simulink model "ABS_v1"  (R2022a)
settings: Solver=VariableStepAuto  StartTime=0.0  StopTime=50.0  RelTol=1e-3
InitFcn:
  | m=75;
  | g=9.81;
  | I=5;
  | R=2;
  | v0=100;
settings Model: Creator=DELL  LastModifiedBy=DELL

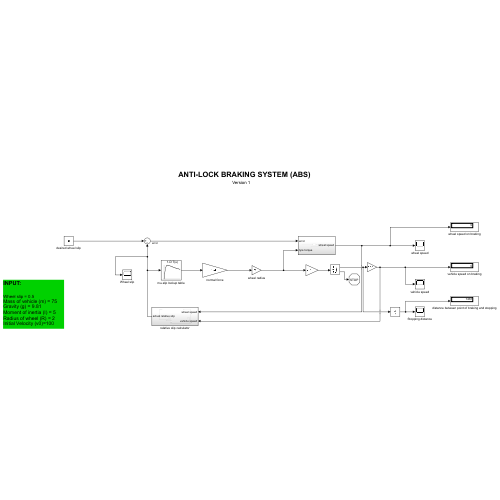
[thumbnail: Simulink's stored preview of the top-level diagram]
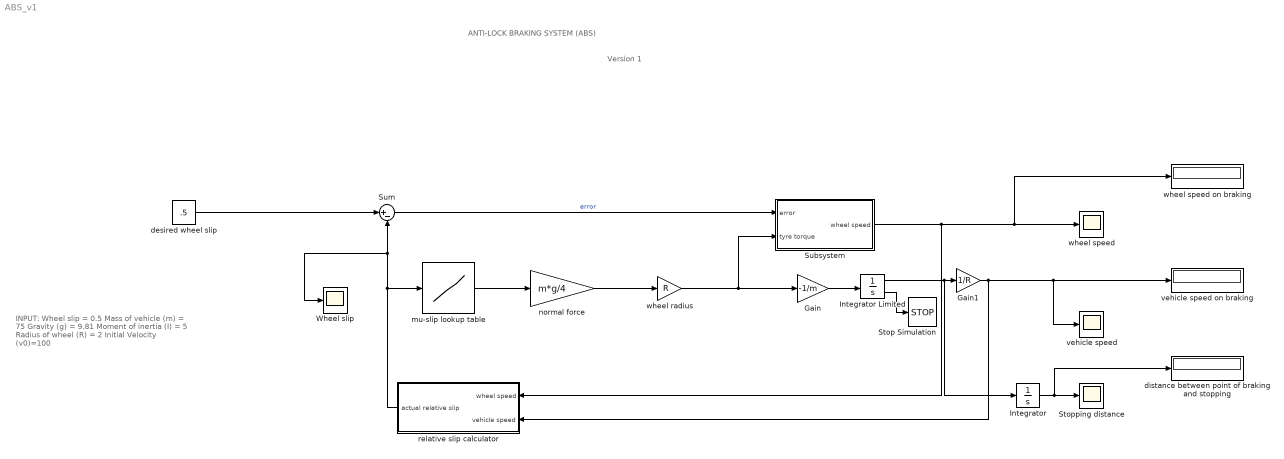
== system ABS_v1 ==
  note: INPUT:
      |
      | Wheel slip = 0.5
      | Mass of vehicle (m) = 75
      | Gravity (g) = 9.81
      | Moment of inertia (I) = 5
      | Radius of wheel (R) = 2
      | Initial Velocity (v0)=100
  note: Version 1
  note: ANTI-LOCK BRAKING SYSTEM (ABS)
  Gain : Gain  Gain=-1/m
  Gain1 : Gain  Gain=1/R
  Integrator : Integrator
  Integrator Limited : Integrator  InitialCondition=v0  LimitOutput=on  UpperSaturationLimit=1000  LowerSaturationLimit=0  ShowSaturationPort=on
  Stop Simulation : Stop
  Stopping distance : Scope
  Subsystem : Subsystem
  Sum : Sum  Inputs=|+-
  Wheel slip : Scope
  desired wheel slip : Constant  Value=.5
  distance between point of braking and stopping : Display
  mu-slip lookup table : Lookup_n-D  NumberOfTableDimensions=1  BreakpointsForDimension1=[0;0.05;0.1;0.15;0.2;0.25;0.3;0.35;0.4;0.45;0.5;0.55;0.6;0.65;0.7;0.75;0.8;0.85;0.9;0.95;1]  Table=[0;0.4;0.8;0.97;1;0.98;0.96;0.94;0.92;0.9;0.88;0.855;0.83;0.81;0.79;0.77;0.75;0.73;0.72;0.71;0.7]  InternalRulePriority=Speed  RndMeth=Simplest
  normal force : Gain  Gain=m*g/4
  relative slip calculator : Subsystem
  vehicle speed : Scope
  vehicle speed on braking : Display
  wheel radius : Gain  Gain=R
  wheel speed : Scope
  wheel speed on braking : Display
  wires:
  desired wheel slip/1 -> Sum/1
  mu-slip lookup table/1 -> normal force/1
  normal force/1 -> wheel radius/1
  Sum/1 -> Subsystem/1(error)  "error"
  wheel radius/1 -> Gain/1, Subsystem/2(tyre torque)
  Gain/1 -> Integrator Limited/1
  Integrator Limited/1 -> Integrator/1, Gain1/1
  Gain1/1 -> relative slip calculator/2(vehicle speed), vehicle speed/1, vehicle speed on braking/1
  Integrator Limited/2 -> Stop Simulation/1
  Integrator/1 -> distance between point of braking and stopping/1, Stopping distance/1
  Subsystem/1(wheel speed) -> wheel speed on braking/1, wheel speed/1, relative slip calculator/1(wheel speed)
  relative slip calculator/1(actual relative slip) -> mu-slip lookup table/1, Wheel slip/1, Sum/2

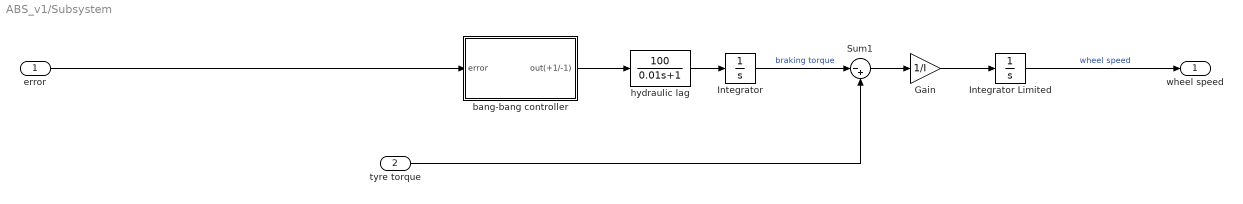
== system ABS_v1/Subsystem ==
  error : Inport
  tyre torque : Inport  Port=2
  Gain : Gain  Gain=1/I
  Integrator : Integrator  LimitOutput=on  UpperSaturationLimit=1000  LowerSaturationLimit=0
  Integrator Limited : Integrator  InitialCondition=v0/R  LimitOutput=on  UpperSaturationLimit=1000  LowerSaturationLimit=0
  Sum1 : Sum  Inputs=|-+
  bang-bang controller : Subsystem
  hydraulic lag : TransferFcn  Numerator=[100]  Denominator=[0.01 1]
  wheel speed : Outport
  wires:
  bang-bang controller/1(out(+1/-1)) -> hydraulic lag/1
  hydraulic lag/1 -> Integrator/1
  Integrator Limited/1 -> wheel speed/1  "wheel speed"
  Sum1/1 -> Gain/1
  error/1 -> bang-bang controller/1(error)
  Integrator/1 -> Sum1/1  "braking torque"
  Gain/1 -> Integrator Limited/1
  tyre torque/1 -> Sum1/2

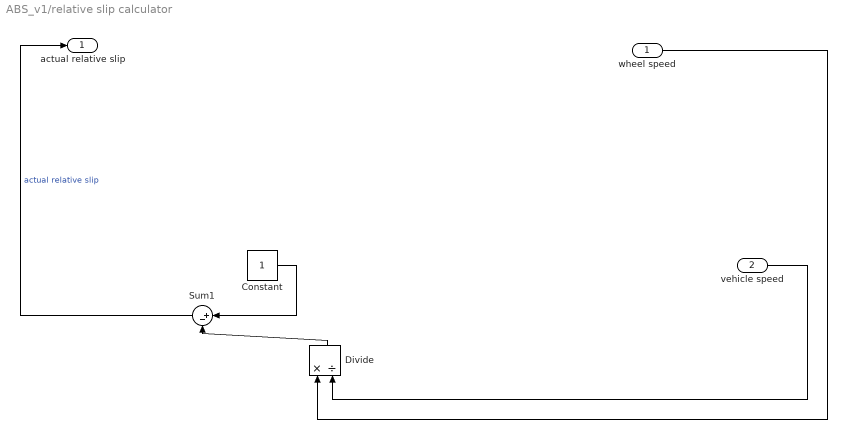
== system ABS_v1/relative slip calculator ==
  wheel speed : Inport
  vehicle speed : Inport  Port=2
  Constant : Constant
  Divide : Product  Inputs=*/
  Sum1 : Sum  Inputs=|+-
  actual relative slip : Outport
  wires:
  Divide/1 -> Sum1/2
  vehicle speed/1 -> Divide/2
  wheel speed/1 -> Divide/1
  Sum1/1 -> actual relative slip/1  "actual relative slip"
  Constant/1 -> Sum1/1

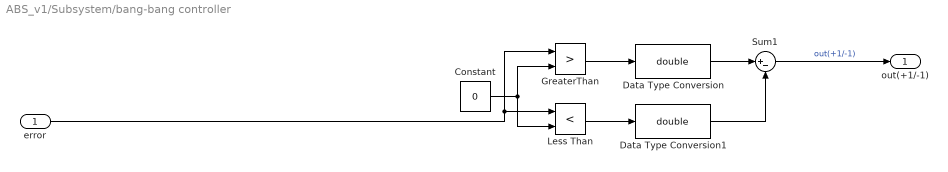
== system ABS_v1/Subsystem/bang-bang controller ==
  error : Inport
  Constant : Constant  Value=0
  Data Type Conversion : DataTypeConversion  OutDataTypeStr=double  SaturateOnIntegerOverflow=off
  Data Type Conversion1 : DataTypeConversion  OutDataTypeStr=double  SaturateOnIntegerOverflow=off
  GreaterThan : RelationalOperator  Operator=>  OutDataTypeStr=boolean  RndMeth=Simplest  InputSameDT=off
  Less Than : RelationalOperator  Operator=<  OutDataTypeStr=boolean  RndMeth=Simplest  InputSameDT=off
  Sum1 : Sum  Inputs=|+-
  out(+1/-1) : Outport
  wires:
  Constant/1 -> Less Than/2, GreaterThan/2
  Data Type Conversion/1 -> Sum1/1
  GreaterThan/1 -> Data Type Conversion/1
  Less Than/1 -> Data Type Conversion1/1
  error/1 -> GreaterThan/1, Less Than/1
  Data Type Conversion1/1 -> Sum1/2
  Sum1/1 -> out(+1/-1)/1  "out(+1/-1)"
